simulink model "NonLinearControlTheoryHW2B"  (R2013a)
settings: Solver=ode45  StartTime=0.0  StopTime=10.0  RelTol=1e-3
settings Model: Creator=Samet  LastModifiedBy=Samet

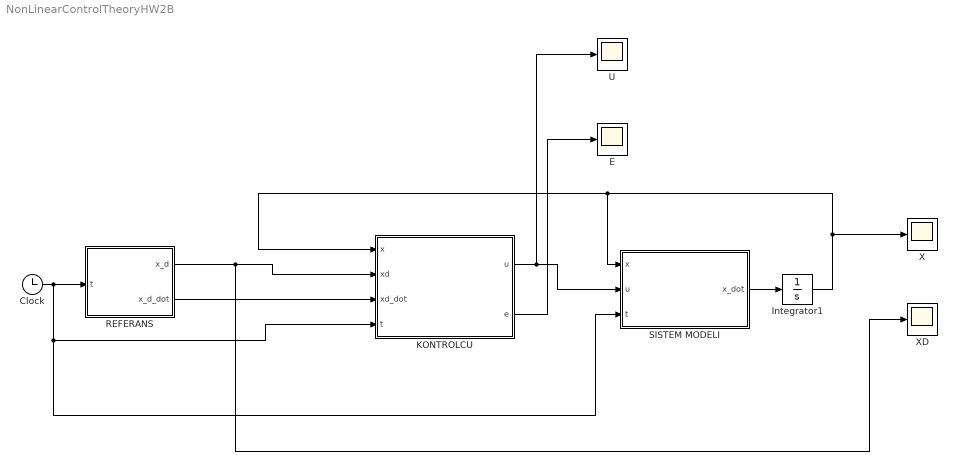
== system NonLinearControlTheoryHW2B ==
  Clock : Clock
  E : Scope
  Integrator1 : Integrator
  KONTROLCU : MATLAB Function  TreatAsAtomicUnit=on
  REFERANS : MATLAB Function  TreatAsAtomicUnit=on
  SISTEM MODELI : MATLAB Function  TreatAsAtomicUnit=on
  U : Scope
      settings: YMax=6
  X : Scope
      settings: YMin=1.2  SaveName=ScopeData2
  XD : Scope
      settings: SaveName=ScopeData3
  wires:
  Clock/1 -> REFERANS/1(t), KONTROLCU/4(t), SISTEM MODELI/3(t)
  SISTEM MODELI/1(x_dot) -> Integrator1/1
  Integrator1/1 -> SISTEM MODELI/1(x), KONTROLCU/1(x), X/1
  KONTROLCU/1(u) -> U/1, SISTEM MODELI/2(u)
  REFERANS/1(x_d) -> XD/1, KONTROLCU/2(xd)
  REFERANS/2(x_d_dot) -> KONTROLCU/3(xd_dot)
  KONTROLCU/2(e) -> E/1

== matlab function NonLinearControlTheoryHW2B/KONTROLCU ==
  data: u output; e output; x input; xd input; xd_dot input; t input
function [u,e]=fcn(x,xd,xd_dot,t)
k=10;
a=5;
b=3;
e=xd-x;
f=-b*x^3+a*sin(t);
u=k*e+xd_dot-f;

== matlab function NonLinearControlTheoryHW2B/REFERANS ==
  data: t input; x_d output; x_d_dot output
function [x_d,x_d_dot] = fcn(t)
x_d = cos(t);
x_d_dot=-sin(t);

== matlab function NonLinearControlTheoryHW2B/SISTEM MODELI ==
  data: x input; u input; x_dot output; t input
function x_dot = fcn(x,u,t)
a=5;
b=3;
x_dot=-b*x^3+a*sin(t)+u;
